simulink model "adc16_mytest"  (R2017a)
settings: Solver=VariableStepDiscrete  StartTime=0.0  StopTime=10.0  RelTol=1e-3
libraries: xbsIndex_r4 x3925, casper_library_misc x8, xps_library x1
(part 1 of 43)
settings Model: Creator=gopal  LastModifiedBy=root
settings DataIOCC: LimitDataPoints=on  SaveFormat=Array
settings OptimizationCC: DefaultParameterBehavior=Inlined  ExpressionDepthLimit=2147483647  LifeSpan=inf
settings DebuggingCC: UnderspecifiedInitializationDetection=Classic  MergeDetectMultiDrivingBlocksExec=none  SolverPrmCheckMsg=warning  StateNameClashWarn=warning  SFUnexpectedBacktrackingDiag=warning  SFNoUnconditionalDefaultTransitionDiag=warning  SFExecutionAtInitializationDiag=none
settings HardwareCC: ProdBitPerPointer=32  ProdBitPerSizeT=32  ProdBitPerPtrDiffT=32  ProdLargestAtomicFloat=None  ProdIntDivRoundTo=Undefined  ProdEndianess=Unspecified  ProdWordSize=32  ProdHWDeviceType=32-bit Generic
settings ModelReferenceCC: PropagateSignalLabelsOutOfModel=off
settings GRTTargetCC: TargetLangStandard=C89/C90 (ANSI)  GeneratePreprocessorConditionals=Disable all
settings ConfigComp: CovMetricSettings=dw  CovHtmlReporting=on  CovSaveCumulativeToWorkspaceVar=on  CovSaveSingleToWorkspaceVar=on  CovExternalEMLEnable=off

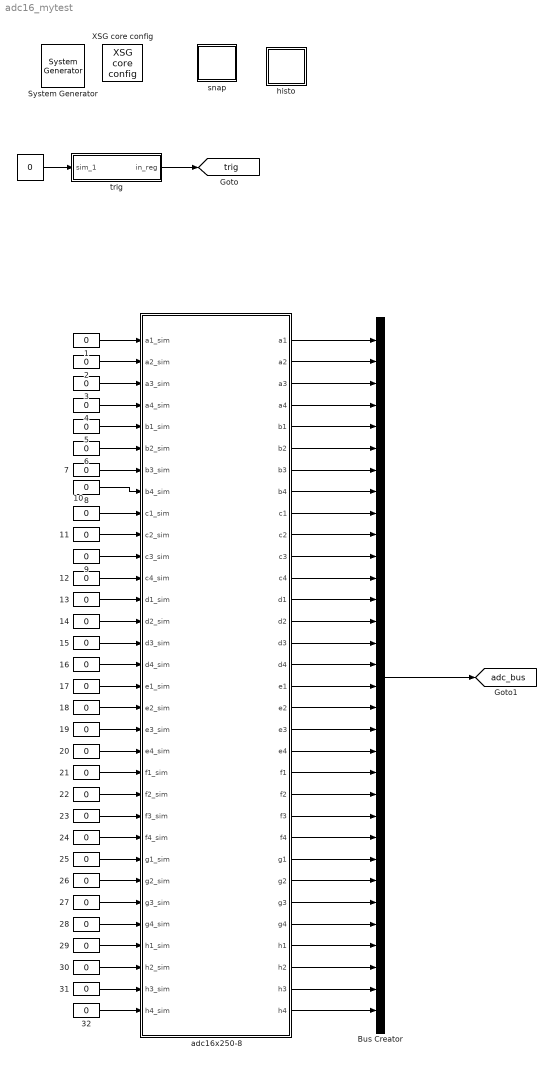
== system adc16_mytest ==
   {,1..32} (33 alike) : Constant  Value=0
  " System Generator" : xbsIndex_r4/ System Generator  Tag=genX  xilinxfamily=virtex6  part=xc6vsx475t  speed=-1  package=ff1759  synthesis_tool=XST  clock_wrapper=Clock Enables  directory=./adc16_mytest/sysgen  proj_type=Project Navigator  Synth_file=XST Defaults  Impl_file=ISE Defaults  testbench=off  simulink_period=1  sysclk_period=4.4444  dcm_input_clock_period=100  incr_netlist=off  trim_vbits=Everywhere in SubSystem  dbl_ovrd=According to Block Masks  core_generation=According to Block Masks  run_coregen=off  deprecated_control=off  eval_field=0  block_type=sysgen
  Bus Creator : BusCreator  Inputs=32
  XSG core config : xps_library/XSG core config  Tag=xps:xsg  hw_sys=ROACH2:sx475t  clk_src=adc0_clk  ROACH_clk_src=sys_clk  ROACH2_clk_src=adc0_clk  MKDIG_clk_src=sys_clk  clk_rate=225  sample_period=1  synthesis_tool=XST
      settings: SourceProductName=CASPER XPS Blockset
  adc16x250-8 : Subsystem  Tag=xps:adc16  AncestorBlock=xps_library/ADCs/adc16x250-8  mask(ADC16){board_count=2, roach2_rev=2, zdok_rev=2}
      mask prompts: board_count "Number of ADC16 Boards"; roach2_rev "ROACH2 Revision"; zdok_rev "ZDOK Pinout Revision"
      mask help: 16-input ADC. When using one ADC16 board, it must be in ZDOK0.
      mask init:
      | % Only board_count is needed by init function
      | adc16_init(gcb, ...
      |     'board_count', board_count);
      settings: AttributesFormatString=r2 rev%<roach2_rev>\nzdok rev%<zdok_rev>
      mask Help:
      | This is the CASPER "yellow block" for the CASPER ADC16 board.  Each ADC
      | board has four ADC chips.  Each ADC chip accepts four inputs.  The four
      | 8-bit outputs from each ADC chip are concatenated into a 32-bit signal.
      mask TypeOptions board_count: 1 | 2
      mask TypeOptions roach2_rev: 1 | 2
      mask TypeOptions zdok_rev: 1 | 2
  histo : Subsystem
  snap : Subsystem
  trig : Subsystem  Tag=xps:sw_reg  AncestorBlock=xps_library/software register  mask(swreg){mode=one value, io_dir=From Processor, io_delay=0, sample_period=1, names=reg, bitwidths=32, arith_types=0, bin_pts=0, sim_port=on, show_format=off}
      mask prompts: io_dir "I/O direction"; io_delay "I/O delay"; sample_period "Sample period"; names "Name:"; bitwidths "Bitwidth:"; arith_types "Type (ufix=0, fix=1, bool=2):"; bin_pts "Binary pt:"; sim_port "Provide sim input/output?"; show_format "Print format string?"
      mask init:
      | swreg_init(gcb)
      settings: AttributesFormatString=1input
      mask TypeOptions mode: one value | fields of equal size | fields of arbitrary size
      mask Callback mode: swreg_cb(gcb);
      mask TypeOptions io_dir: To Processor | From Processor
      mask Callback io_dir:
      | mask_enables = get_param(gcb, 'MaskEnables');
      | mask_names = get_param(gcb, 'MaskNames');
      | if strcmp(get_param(gcb, 'io_dir'), 'To Processor'),
      |     mask_enables{ismember(mask_names, 'sample_period')} = 'off';
      | else
      |     mask_enables{ismember(mask_names, 'sample_period')} = 'on';
      | end
      | set_param(gcb, 'MaskEnables', mask_enables);
      mask Callback bitwidths: swreg_maskcheck(gcb);
      mask Callback arith_types: [numios, ~, ~, ~, current_types] = swreg_maskcheck(gcb);
      mask Callback bin_pts: swreg_maskcheck(gcb);
  tag scope: adc_bus=global, trig=global
  wires:
  " "/1 -> trig/1(sim_1)
  trig/1(in_reg) -> [trig]
  " 1"/1 -> adc16x250-8/1(a1_sim)
  " 13"/1 -> adc16x250-8/13(d1_sim)
  " 4"/1 -> adc16x250-8/4(a4_sim)
  " 12"/1 -> adc16x250-8/12(c4_sim)
  " 6"/1 -> adc16x250-8/6(b2_sim)
  " 2"/1 -> adc16x250-8/2(a2_sim)
  " 15"/1 -> adc16x250-8/15(d3_sim)
  " 9"/1 -> adc16x250-8/11(c3_sim)
  " 5"/1 -> adc16x250-8/5(b1_sim)
  " 16"/1 -> adc16x250-8/16(d4_sim)
  " 7"/1 -> adc16x250-8/7(b3_sim)
  " 11"/1 -> adc16x250-8/10(c2_sim)
  " 10"/1 -> adc16x250-8/9(c1_sim)
  " 14"/1 -> adc16x250-8/14(d2_sim)
  " 29"/1 -> adc16x250-8/29(h1_sim)
  " 27"/1 -> adc16x250-8/27(g3_sim)
  " 18"/1 -> adc16x250-8/18(e2_sim)
  " 17"/1 -> adc16x250-8/17(e1_sim)
  " 19"/1 -> adc16x250-8/19(e3_sim)
  " 26"/1 -> adc16x250-8/26(g2_sim)
  " 20"/1 -> adc16x250-8/20(e4_sim)
  " 21"/1 -> adc16x250-8/21(f1_sim)
  " 24"/1 -> adc16x250-8/24(f4_sim)
  " 28"/1 -> adc16x250-8/28(g4_sim)
  " 23"/1 -> adc16x250-8/23(f3_sim)
  " 22"/1 -> adc16x250-8/22(f2_sim)
  " 31"/1 -> adc16x250-8/31(h3_sim)
  " 25"/1 -> adc16x250-8/25(g1_sim)
  " 30"/1 -> adc16x250-8/30(h2_sim)
  " 32"/1 -> adc16x250-8/32(h4_sim)
  " 3"/1 -> adc16x250-8/3(a3_sim)
  " 8"/1 -> adc16x250-8/8(b4_sim)
  adc16x250-8/14(d2) -> Bus Creator/14
  adc16x250-8/15(d3) -> Bus Creator/15
  adc16x250-8/16(d4) -> Bus Creator/16
  adc16x250-8/10(c2) -> Bus Creator/10
  adc16x250-8/1(a1) -> Bus Creator/1
  adc16x250-8/2(a2) -> Bus Creator/2
  adc16x250-8/3(a3) -> Bus Creator/3
  adc16x250-8/4(a4) -> Bus Creator/4
  adc16x250-8/5(b1) -> Bus Creator/5
  adc16x250-8/6(b2) -> Bus Creator/6
  adc16x250-8/7(b3) -> Bus Creator/7
  adc16x250-8/8(b4) -> Bus Creator/8
  adc16x250-8/9(c1) -> Bus Creator/9
  adc16x250-8/11(c3) -> Bus Creator/11
  adc16x250-8/12(c4) -> Bus Creator/12
  adc16x250-8/13(d1) -> Bus Creator/13
  adc16x250-8/22(f2) -> Bus Creator/22
  adc16x250-8/20(e4) -> Bus Creator/20
  adc16x250-8/21(f1) -> Bus Creator/21
  adc16x250-8/19(e3) -> Bus Creator/19
  adc16x250-8/25(g1) -> Bus Creator/25
  adc16x250-8/23(f3) -> Bus Creator/23
  adc16x250-8/18(e2) -> Bus Creator/18
  adc16x250-8/17(e1) -> Bus Creator/17
  adc16x250-8/24(f4) -> Bus Creator/24
  adc16x250-8/26(g2) -> Bus Creator/26
  adc16x250-8/27(g3) -> Bus Creator/27
  adc16x250-8/28(g4) -> Bus Creator/28
  adc16x250-8/29(h1) -> Bus Creator/29
  adc16x250-8/32(h4) -> Bus Creator/32
  adc16x250-8/30(h2) -> Bus Creator/30
  adc16x250-8/31(h3) -> Bus Creator/31
  Bus Creator/1 -> [adc_bus]

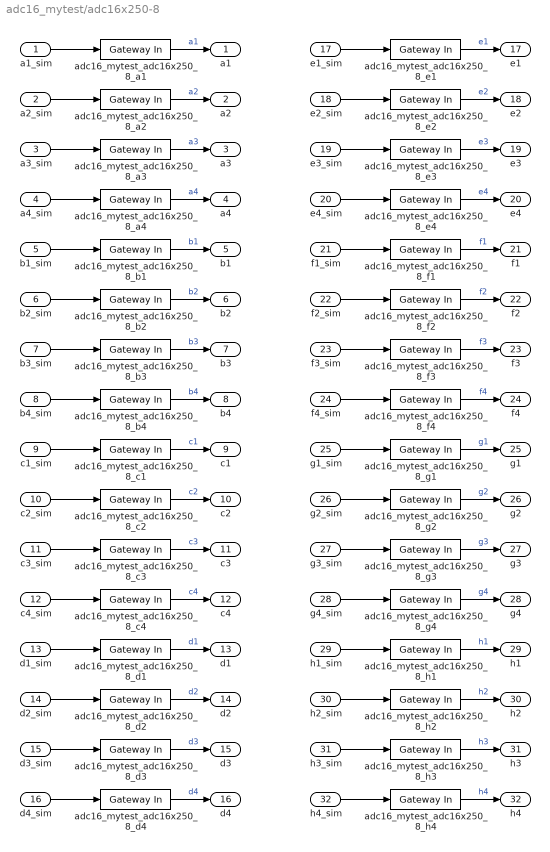
== system adc16_mytest/adc16x250-8 ==
  a1_sim : Inport
  a2_sim : Inport  Port=2
  a3_sim : Inport  Port=3
  a4_sim : Inport  Port=4
  b1_sim : Inport  Port=5
  b2_sim : Inport  Port=6
  b3_sim : Inport  Port=7
  b4_sim : Inport  Port=8
  c1_sim : Inport  Port=9
  c2_sim : Inport  Port=10
  c3_sim : Inport  Port=11
  c4_sim : Inport  Port=12
  d1_sim : Inport  Port=13
  d2_sim : Inport  Port=14
  d3_sim : Inport  Port=15
  d4_sim : Inport  Port=16
  e1_sim : Inport  Port=17
  e2_sim : Inport  Port=18
  e3_sim : Inport  Port=19
  e4_sim : Inport  Port=20
  f1_sim : Inport  Port=21
  f2_sim : Inport  Port=22
  f3_sim : Inport  Port=23
  f4_sim : Inport  Port=24
  g1_sim : Inport  Port=25
  g2_sim : Inport  Port=26
  g3_sim : Inport  Port=27
  g4_sim : Inport  Port=28
  h1_sim : Inport  Port=29
  h2_sim : Inport  Port=30
  h3_sim : Inport  Port=31
  h4_sim : Inport  Port=32
  adc16_mytest_adc16x250_8_a{1..4} (4 alike) : xbsIndex_r4/Gateway In  gui_display_data_type=Fixed-point  arith_type="Signed  (2's comp)"  n_bits=8  bin_pt=7  preci_type=Single  exp_width=8  frac_width=24  quantization="Round  (unbiased: +/- Inf)"  overflow=Saturate  period=1  dbl_ovrd=off  timing_constraint=None  locs_specified=off  LOCs={}  UseAsADC=off  ADCChannel='1'  inherit_from_input=off  hdl_port=on  block_type=gatewayin
  adc16_mytest_adc16x250_8_b{1..4} (4 alike) : xbsIndex_r4/Gateway In  gui_display_data_type=Fixed-point  arith_type="Signed  (2's comp)"  n_bits=8  bin_pt=7  preci_type=Single  exp_width=8  frac_width=24  quantization="Round  (unbiased: +/- Inf)"  overflow=Saturate  period=1  dbl_ovrd=off  timing_constraint=None  locs_specified=off  LOCs={}  UseAsADC=off  ADCChannel='1'  inherit_from_input=off  hdl_port=on  block_type=gatewayin
  adc16_mytest_adc16x250_8_c{1..4} (4 alike) : xbsIndex_r4/Gateway In  gui_display_data_type=Fixed-point  arith_type="Signed  (2's comp)"  n_bits=8  bin_pt=7  preci_type=Single  exp_width=8  frac_width=24  quantization="Round  (unbiased: +/- Inf)"  overflow=Saturate  period=1  dbl_ovrd=off  timing_constraint=None  locs_specified=off  LOCs={}  UseAsADC=off  ADCChannel='1'  inherit_from_input=off  hdl_port=on  block_type=gatewayin
  adc16_mytest_adc16x250_8_d{1..4} (4 alike) : xbsIndex_r4/Gateway In  gui_display_data_type=Fixed-point  arith_type="Signed  (2's comp)"  n_bits=8  bin_pt=7  preci_type=Single  exp_width=8  frac_width=24  quantization="Round  (unbiased: +/- Inf)"  overflow=Saturate  period=1  dbl_ovrd=off  timing_constraint=None  locs_specified=off  LOCs={}  UseAsADC=off  ADCChannel='1'  inherit_from_input=off  hdl_port=on  block_type=gatewayin
  adc16_mytest_adc16x250_8_e{1..4} (4 alike) : xbsIndex_r4/Gateway In  gui_display_data_type=Fixed-point  arith_type="Signed  (2's comp)"  n_bits=8  bin_pt=7  preci_type=Single  exp_width=8  frac_width=24  quantization="Round  (unbiased: +/- Inf)"  overflow=Saturate  period=1  dbl_ovrd=off  timing_constraint=None  locs_specified=off  LOCs={}  UseAsADC=off  ADCChannel='1'  inherit_from_input=off  hdl_port=on  block_type=gatewayin
  adc16_mytest_adc16x250_8_f{1..4} (4 alike) : xbsIndex_r4/Gateway In  gui_display_data_type=Fixed-point  arith_type="Signed  (2's comp)"  n_bits=8  bin_pt=7  preci_type=Single  exp_width=8  frac_width=24  quantization="Round  (unbiased: +/- Inf)"  overflow=Saturate  period=1  dbl_ovrd=off  timing_constraint=None  locs_specified=off  LOCs={}  UseAsADC=off  ADCChannel='1'  inherit_from_input=off  hdl_port=on  block_type=gatewayin
  adc16_mytest_adc16x250_8_g{1..4} (4 alike) : xbsIndex_r4/Gateway In  gui_display_data_type=Fixed-point  arith_type="Signed  (2's comp)"  n_bits=8  bin_pt=7  preci_type=Single  exp_width=8  frac_width=24  quantization="Round  (unbiased: +/- Inf)"  overflow=Saturate  period=1  dbl_ovrd=off  timing_constraint=None  locs_specified=off  LOCs={}  UseAsADC=off  ADCChannel='1'  inherit_from_input=off  hdl_port=on  block_type=gatewayin
  adc16_mytest_adc16x250_8_h{1..4} (4 alike) : xbsIndex_r4/Gateway In  gui_display_data_type=Fixed-point  arith_type="Signed  (2's comp)"  n_bits=8  bin_pt=7  preci_type=Single  exp_width=8  frac_width=24  quantization="Round  (unbiased: +/- Inf)"  overflow=Saturate  period=1  dbl_ovrd=off  timing_constraint=None  locs_specified=off  LOCs={}  UseAsADC=off  ADCChannel='1'  inherit_from_input=off  hdl_port=on  block_type=gatewayin
  a1 : Outport
  a2 : Outport  Port=2
  a3 : Outport  Port=3
  a4 : Outport  Port=4
  b1 : Outport  Port=5
  b2 : Outport  Port=6
  b3 : Outport  Port=7
  b4 : Outport  Port=8
  c1 : Outport  Port=9
  c2 : Outport  Port=10
  c3 : Outport  Port=11
  c4 : Outport  Port=12
  d1 : Outport  Port=13
  d2 : Outport  Port=14
  d3 : Outport  Port=15
  d4 : Outport  Port=16
  e1 : Outport  Port=17
  e2 : Outport  Port=18
  e3 : Outport  Port=19
  e4 : Outport  Port=20
  f1 : Outport  Port=21
  f2 : Outport  Port=22
  f3 : Outport  Port=23
  f4 : Outport  Port=24
  g1 : Outport  Port=25
  g2 : Outport  Port=26
  g3 : Outport  Port=27
  g4 : Outport  Port=28
  h1 : Outport  Port=29
  h2 : Outport  Port=30
  h3 : Outport  Port=31
  h4 : Outport  Port=32
  wires:
  a1_sim/1 -> adc16_mytest_adc16x250_8_a1/1
  adc16_mytest_adc16x250_8_a1/1 -> a1/1  "a1"
  a2_sim/1 -> adc16_mytest_adc16x250_8_a2/1
  adc16_mytest_adc16x250_8_a2/1 -> a2/1  "a2"
  a3_sim/1 -> adc16_mytest_adc16x250_8_a3/1
  adc16_mytest_adc16x250_8_a3/1 -> a3/1  "a3"
  a4_sim/1 -> adc16_mytest_adc16x250_8_a4/1
  adc16_mytest_adc16x250_8_a4/1 -> a4/1  "a4"
  b1_sim/1 -> adc16_mytest_adc16x250_8_b1/1
  adc16_mytest_adc16x250_8_b1/1 -> b1/1  "b1"
  b2_sim/1 -> adc16_mytest_adc16x250_8_b2/1
  adc16_mytest_adc16x250_8_b2/1 -> b2/1  "b2"
  b3_sim/1 -> adc16_mytest_adc16x250_8_b3/1
  adc16_mytest_adc16x250_8_b3/1 -> b3/1  "b3"
  b4_sim/1 -> adc16_mytest_adc16x250_8_b4/1
  adc16_mytest_adc16x250_8_b4/1 -> b4/1  "b4"
  c1_sim/1 -> adc16_mytest_adc16x250_8_c1/1
  adc16_mytest_adc16x250_8_c1/1 -> c1/1  "c1"
  c2_sim/1 -> adc16_mytest_adc16x250_8_c2/1
  adc16_mytest_adc16x250_8_c2/1 -> c2/1  "c2"
  c3_sim/1 -> adc16_mytest_adc16x250_8_c3/1
  adc16_mytest_adc16x250_8_c3/1 -> c3/1  "c3"
  c4_sim/1 -> adc16_mytest_adc16x250_8_c4/1
  adc16_mytest_adc16x250_8_c4/1 -> c4/1  "c4"
  d1_sim/1 -> adc16_mytest_adc16x250_8_d1/1
  adc16_mytest_adc16x250_8_d1/1 -> d1/1  "d1"
  d2_sim/1 -> adc16_mytest_adc16x250_8_d2/1
  adc16_mytest_adc16x250_8_d2/1 -> d2/1  "d2"
  d3_sim/1 -> adc16_mytest_adc16x250_8_d3/1
  adc16_mytest_adc16x250_8_d3/1 -> d3/1  "d3"
  d4_sim/1 -> adc16_mytest_adc16x250_8_d4/1
  adc16_mytest_adc16x250_8_d4/1 -> d4/1  "d4"
  e1_sim/1 -> adc16_mytest_adc16x250_8_e1/1
  adc16_mytest_adc16x250_8_e1/1 -> e1/1  "e1"
  e2_sim/1 -> adc16_mytest_adc16x250_8_e2/1
  adc16_mytest_adc16x250_8_e2/1 -> e2/1  "e2"
  e3_sim/1 -> adc16_mytest_adc16x250_8_e3/1
  adc16_mytest_adc16x250_8_e3/1 -> e3/1  "e3"
  e4_sim/1 -> adc16_mytest_adc16x250_8_e4/1
  adc16_mytest_adc16x250_8_e4/1 -> e4/1  "e4"
  f1_sim/1 -> adc16_mytest_adc16x250_8_f1/1
  adc16_mytest_adc16x250_8_f1/1 -> f1/1  "f1"
  f2_sim/1 -> adc16_mytest_adc16x250_8_f2/1
  adc16_mytest_adc16x250_8_f2/1 -> f2/1  "f2"
  f3_sim/1 -> adc16_mytest_adc16x250_8_f3/1
  adc16_mytest_adc16x250_8_f3/1 -> f3/1  "f3"
  f4_sim/1 -> adc16_mytest_adc16x250_8_f4/1
  adc16_mytest_adc16x250_8_f4/1 -> f4/1  "f4"
  g1_sim/1 -> adc16_mytest_adc16x250_8_g1/1
  adc16_mytest_adc16x250_8_g1/1 -> g1/1  "g1"
  g2_sim/1 -> adc16_mytest_adc16x250_8_g2/1
  adc16_mytest_adc16x250_8_g2/1 -> g2/1  "g2"
  g3_sim/1 -> adc16_mytest_adc16x250_8_g3/1
  adc16_mytest_adc16x250_8_g3/1 -> g3/1  "g3"
  g4_sim/1 -> adc16_mytest_adc16x250_8_g4/1
  adc16_mytest_adc16x250_8_g4/1 -> g4/1  "g4"
  h1_sim/1 -> adc16_mytest_adc16x250_8_h1/1
  adc16_mytest_adc16x250_8_h1/1 -> h1/1  "h1"
  h2_sim/1 -> adc16_mytest_adc16x250_8_h2/1
  adc16_mytest_adc16x250_8_h2/1 -> h2/1  "h2"
  h3_sim/1 -> adc16_mytest_adc16x250_8_h3/1
  adc16_mytest_adc16x250_8_h3/1 -> h3/1  "h3"
  h4_sim/1 -> adc16_mytest_adc16x250_8_h4/1
  adc16_mytest_adc16x250_8_h4/1 -> h4/1  "h4"

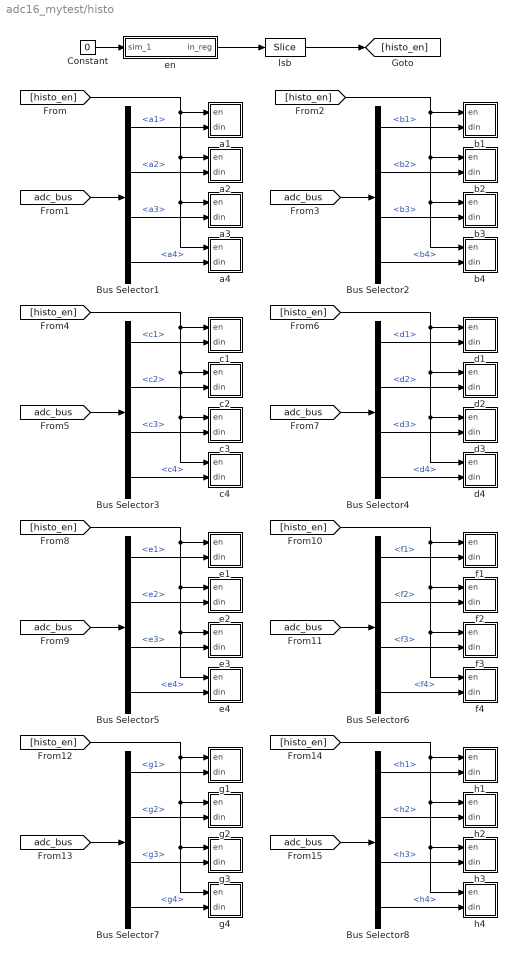
== system adc16_mytest/histo ==
  Bus Selector1 : BusSelector  OutputSignals=a1,a2,a3,a4
  Bus Selector2 : BusSelector  OutputSignals=b1,b2,b3,b4
  Bus Selector3 : BusSelector  OutputSignals=c1,c2,c3,c4
  Bus Selector4 : BusSelector  OutputSignals=d1,d2,d3,d4
  Bus Selector5 : BusSelector  OutputSignals=e1,e2,e3,e4
  Bus Selector6 : BusSelector  OutputSignals=f1,f2,f3,f4
  Bus Selector7 : BusSelector  OutputSignals=g1,g2,g3,g4
  Bus Selector8 : BusSelector  OutputSignals=h1,h2,h3,h4
  Constant : Constant  Value=0
  a1 : Subsystem
  a2 : Subsystem
  a3 : Subsystem
  a4 : Subsystem
  b1 : Subsystem
  b2 : Subsystem
  b3 : Subsystem
  b4 : Subsystem
  c1 : Subsystem
  c2 : Subsystem
  c3 : Subsystem
  c4 : Subsystem
  d1 : Subsystem
  d2 : Subsystem
  d3 : Subsystem
  d4 : Subsystem
  e1 : Subsystem
  e2 : Subsystem
  e3 : Subsystem
  e4 : Subsystem
  en : Subsystem  Tag=xps:sw_reg  AncestorBlock=xps_library/software register  mask(swreg){mode=one value, io_dir=From Processor, io_delay=0, sample_period=1, names=reg, bitwidths=32, arith_types=0, bin_pts=0, sim_port=on, show_format=off}
      mask prompts: io_dir "I/O direction"; io_delay "I/O delay"; sample_period "Sample period"; names "Name:"; bitwidths "Bitwidth:"; arith_types "Type (ufix=0, fix=1, bool=2):"; bin_pts "Binary pt:"; sim_port "Provide sim input/output?"; show_format "Print format string?"
      mask init:
      | swreg_init(gcb)
      settings: AttributesFormatString=1input
      mask TypeOptions mode: one value | fields of equal size | fields of arbitrary size
      mask Callback mode: swreg_cb(gcb);
      mask TypeOptions io_dir: To Processor | From Processor
      mask Callback io_dir:
      | mask_enables = get_param(gcb, 'MaskEnables');
      | mask_names = get_param(gcb, 'MaskNames');
      | if strcmp(get_param(gcb, 'io_dir'), 'To Processor'),
      |     mask_enables{ismember(mask_names, 'sample_period')} = 'off';
      | else
      |     mask_enables{ismember(mask_names, 'sample_period')} = 'on';
      | end
      | set_param(gcb, 'MaskEnables', mask_enables);
      mask Callback bitwidths: swreg_maskcheck(gcb);
      mask Callback arith_types: [numios, ~, ~, ~, current_types] = swreg_maskcheck(gcb);
      mask Callback bin_pts: swreg_maskcheck(gcb);
  f1 : Subsystem
  f2 : Subsystem
  f3 : Subsystem
  f4 : Subsystem
  g1 : Subsystem
  g2 : Subsystem
  g3 : Subsystem
  g4 : Subsystem
  h1 : Subsystem
  h2 : Subsystem
  h3 : Subsystem
  h4 : Subsystem
  lsb : xbsIndex_r4/Slice  nbits=1  boolean_output=on  mode=Lower Bit Location + Width  bit1=0  base1=MSB of Input  bit0=0  base0=LSB of Input  dbl_ovrd=off  block_type=slice
  wires:
  Bus Selector8/2 -> h2/2(din)  "<h2>"
  Bus Selector8/3 -> h3/2(din)  "<h3>"
  Bus Selector8/4 -> h4/2(din)  "<h4>"
  Bus Selector8/1 -> h1/2(din)  "<h1>"
  [histo_en] -> h1/1(en), h2/1(en), h3/1(en), h4/1(en)
  [adc_bus] -> Bus Selector8/1
  Bus Selector7/2 -> g2/2(din)  "<g2>"
  Bus Selector7/3 -> g3/2(din)  "<g3>"
  Bus Selector7/4 -> g4/2(din)  "<g4>"
  Bus Selector7/1 -> g1/2(din)  "<g1>"
  [histo_en] -> g1/1(en), g2/1(en), g3/1(en), g4/1(en)
  [adc_bus] -> Bus Selector7/1
  Bus Selector6/2 -> f2/2(din)  "<f2>"
  Bus Selector6/3 -> f3/2(din)  "<f3>"
  Bus Selector6/4 -> f4/2(din)  "<f4>"
  Bus Selector6/1 -> f1/2(din)  "<f1>"
  [histo_en] -> f1/1(en), f2/1(en), f3/1(en), f4/1(en)
  [adc_bus] -> Bus Selector6/1
  Bus Selector5/2 -> e2/2(din)  "<e2>"
  Bus Selector5/3 -> e3/2(din)  "<e3>"
  Bus Selector5/4 -> e4/2(din)  "<e4>"
  Bus Selector5/1 -> e1/2(din)  "<e1>"
  [histo_en] -> e1/1(en), e2/1(en), e3/1(en), e4/1(en)
  [adc_bus] -> Bus Selector5/1
  Bus Selector4/2 -> d2/2(din)  "<d2>"
  Bus Selector4/3 -> d3/2(din)  "<d3>"
  Bus Selector4/4 -> d4/2(din)  "<d4>"
  Bus Selector4/1 -> d1/2(din)  "<d1>"
  [histo_en] -> d1/1(en), d2/1(en), d3/1(en), d4/1(en)
  [adc_bus] -> Bus Selector4/1
  Bus Selector3/2 -> c2/2(din)  "<c2>"
  Bus Selector3/3 -> c3/2(din)  "<c3>"
  Bus Selector3/4 -> c4/2(din)  "<c4>"
  Bus Selector3/1 -> c1/2(din)  "<c1>"
  [histo_en] -> c1/1(en), c2/1(en), c3/1(en), c4/1(en)
  [adc_bus] -> Bus Selector3/1
  Bus Selector2/2 -> b2/2(din)  "<b2>"
  Bus Selector2/3 -> b3/2(din)  "<b3>"
  Bus Selector2/4 -> b4/2(din)  "<b4>"
  Bus Selector2/1 -> b1/2(din)  "<b1>"
  [histo_en] -> b1/1(en), b2/1(en), b3/1(en), b4/1(en)
  [adc_bus] -> Bus Selector2/1
  Bus Selector1/2 -> a2/2(din)  "<a2>"
  Bus Selector1/3 -> a3/2(din)  "<a3>"
  Bus Selector1/4 -> a4/2(din)  "<a4>"
  Bus Selector1/1 -> a1/2(din)  "<a1>"
  [histo_en] -> a1/1(en), a2/1(en), a3/1(en), a4/1(en)
  [adc_bus] -> Bus Selector1/1
  lsb/1 -> [histo_en]
  Constant/1 -> en/1(sim_1)
  en/1(in_reg) -> lsb/1

== system adc16_mytest/snap ==
  BitBasher : xbsIndex_r4/BitBasher  bitexpr=|  display_expr=off  sr_1=1  arith_type1=Unsigned  bin_pt1=0  sr_2=2  arith_type2=Unsigned  bin_pt2=0  sr_3=3  arith_type3=Unsigned  bin_pt3=0  sr_4=4  arith_type4=Unsigned  bin_pt4=0  dbl_ovrd=off  block_type=bitbasher
      | <!DOCTYPE HTML PUBLIC "-//W3C//DTD HTML 4.0//EN" "http://www.w3.org/TR/REC-html40/strict.dtd">
      | <html><head><meta name="qrichtext" content="1" /><style type="text/css">
      | p, li { white-space: pre-wrap; }
      | </style></head><body style=" font-family:'Sans'; font-size:10pt; font-weight:400; font-style:normal;">
      | <p style=" margin-top:12px; margin-bottom:12px; margin-left:0px; margin-right:0px; -qt-block-indent:0; text-indent:0px;"><span style=" font-family:'MS Shell Dlg'; font-size:8pt;">o={p1,p2,p3,p4}</span></p></body></html>
  BitBasher1 : xbsIndex_r4/BitBasher  bitexpr=|  display_expr=off  sr_1=1  arith_type1=Unsigned  bin_pt1=0  sr_2=2  arith_type2=Unsigned  bin_pt2=0  sr_3=3  arith_type3=Unsigned  bin_pt3=0  sr_4=4  arith_type4=Unsigned  bin_pt4=0  dbl_ovrd=off  block_type=bitbasher
      | <!DOCTYPE HTML PUBLIC "-//W3C//DTD HTML 4.0//EN" "http://www.w3.org/TR/REC-html40/strict.dtd">
      | <html><head><meta name="qrichtext" content="1" /><style type="text/css">
      | p, li { white-space: pre-wrap; }
      | </style></head><body style=" font-family:'Sans'; font-size:10pt; font-weight:400; font-style:normal;">
      | <p style=" margin-top:12px; margin-bottom:12px; margin-left:0px; margin-right:0px; -qt-block-indent:0; text-indent:0px;"><span style=" font-family:'MS Shell Dlg'; font-size:8pt;">o={p1,p2,p3,p4}</span></p></body></html>
  BitBasher10 : xbsIndex_r4/BitBasher  bitexpr=|  display_expr=off  sr_1=1  arith_type1=Unsigned  bin_pt1=0  sr_2=2  arith_type2=Unsigned  bin_pt2=0  sr_3=3  arith_type3=Unsigned  bin_pt3=0  sr_4=4  arith_type4=Unsigned  bin_pt4=0  dbl_ovrd=off  block_type=bitbasher
      | <!DOCTYPE HTML PUBLIC "-//W3C//DTD HTML 4.0//EN" "http://www.w3.org/TR/REC-html40/strict.dtd">
      | <html><head><meta name="qrichtext" content="1" /><style type="text/css">
      | p, li { white-space: pre-wrap; }
      | </style></head><body style=" font-family:'Sans'; font-size:10pt; font-weight:400; font-style:normal;">
      | <p style=" margin-top:12px; margin-bottom:12px; margin-left:0px; margin-right:0px; -qt-block-indent:0; text-indent:0px;"><span style=" font-family:'MS Shell Dlg'; font-size:8pt;">o={p1,p2,p3,p4}</span></p></body></html>
  BitBasher11 : xbsIndex_r4/BitBasher  bitexpr=|  display_expr=off  sr_1=1  arith_type1=Unsigned  bin_pt1=0  sr_2=2  arith_type2=Unsigned  bin_pt2=0  sr_3=3  arith_type3=Unsigned  bin_pt3=0  sr_4=4  arith_type4=Unsigned  bin_pt4=0  dbl_ovrd=off  block_type=bitbasher
      | <!DOCTYPE HTML PUBLIC "-//W3C//DTD HTML 4.0//EN" "http://www.w3.org/TR/REC-html40/strict.dtd">
      | <html><head><meta name="qrichtext" content="1" /><style type="text/css">
      | p, li { white-space: pre-wrap; }
      | </style></head><body style=" font-family:'Sans'; font-size:10pt; font-weight:400; font-style:normal;">
      | <p style=" margin-top:12px; margin-bottom:12px; margin-left:0px; margin-right:0px; -qt-block-indent:0; text-indent:0px;"><span style=" font-family:'MS Shell Dlg'; font-size:8pt;">o={p1,p2,p3,p4}</span></p></body></html>
  BitBasher2 : xbsIndex_r4/BitBasher  bitexpr=|  display_expr=off  sr_1=1  arith_type1=Unsigned  bin_pt1=0  sr_2=2  arith_type2=Unsigned  bin_pt2=0  sr_3=3  arith_type3=Unsigned  bin_pt3=0  sr_4=4  arith_type4=Unsigned  bin_pt4=0  dbl_ovrd=off  block_type=bitbasher
      | <!DOCTYPE HTML PUBLIC "-//W3C//DTD HTML 4.0//EN" "http://www.w3.org/TR/REC-html40/strict.dtd">
      | <html><head><meta name="qrichtext" content="1" /><style type="text/css">
      | p, li { white-space: pre-wrap; }
      | </style></head><body style=" font-family:'Sans'; font-size:10pt; font-weight:400; font-style:normal;">
      | <p style=" margin-top:12px; margin-bottom:12px; margin-left:0px; margin-right:0px; -qt-block-indent:0; text-indent:0px;"><span style=" font-family:'MS Shell Dlg'; font-size:8pt;">o={p1,p2,p3,p4}</span></p></body></html>
  BitBasher3 : xbsIndex_r4/BitBasher  bitexpr=|  display_expr=off  sr_1=1  arith_type1=Unsigned  bin_pt1=0  sr_2=2  arith_type2=Unsigned  bin_pt2=0  sr_3=3  arith_type3=Unsigned  bin_pt3=0  sr_4=4  arith_type4=Unsigned  bin_pt4=0  dbl_ovrd=off  block_type=bitbasher
      | <!DOCTYPE HTML PUBLIC "-//W3C//DTD HTML 4.0//EN" "http://www.w3.org/TR/REC-html40/strict.dtd">
      | <html><head><meta name="qrichtext" content="1" /><style type="text/css">
      | p, li { white-space: pre-wrap; }
      | </style></head><body style=" font-family:'Sans'; font-size:10pt; font-weight:400; font-style:normal;">
      | <p style=" margin-top:12px; margin-bottom:12px; margin-left:0px; margin-right:0px; -qt-block-indent:0; text-indent:0px;"><span style=" font-family:'MS Shell Dlg'; font-size:8pt;">o={p1,p2,p3,p4}</span></p></body></html>
  BitBasher8 : xbsIndex_r4/BitBasher  bitexpr=|  display_expr=off  sr_1=1  arith_type1=Unsigned  bin_pt1=0  sr_2=2  arith_type2=Unsigned  bin_pt2=0  sr_3=3  arith_type3=Unsigned  bin_pt3=0  sr_4=4  arith_type4=Unsigned  bin_pt4=0  dbl_ovrd=off  block_type=bitbasher
      | <!DOCTYPE HTML PUBLIC "-//W3C//DTD HTML 4.0//EN" "http://www.w3.org/TR/REC-html40/strict.dtd">
      | <html><head><meta name="qrichtext" content="1" /><style type="text/css">
      | p, li { white-space: pre-wrap; }
      | </style></head><body style=" font-family:'Sans'; font-size:10pt; font-weight:400; font-style:normal;">
      | <p style=" margin-top:12px; margin-bottom:12px; margin-left:0px; margin-right:0px; -qt-block-indent:0; text-indent:0px;"><span style=" font-family:'MS Shell Dlg'; font-size:8pt;">o={p1,p2,p3,p4}</span></p></body></html>
  BitBasher9 : xbsIndex_r4/BitBasher  bitexpr=|  display_expr=off  sr_1=1  arith_type1=Unsigned  bin_pt1=0  sr_2=2  arith_type2=Unsigned  bin_pt2=0  sr_3=3  arith_type3=Unsigned  bin_pt3=0  sr_4=4  arith_type4=Unsigned  bin_pt4=0  dbl_ovrd=off  block_type=bitbasher
      | <!DOCTYPE HTML PUBLIC "-//W3C//DTD HTML 4.0//EN" "http://www.w3.org/TR/REC-html40/strict.dtd">
      | <html><head><meta name="qrichtext" content="1" /><style type="text/css">
      | p, li { white-space: pre-wrap; }
      | </style></head><body style=" font-family:'Sans'; font-size:10pt; font-weight:400; font-style:normal;">
      | <p style=" margin-top:12px; margin-bottom:12px; margin-left:0px; margin-right:0px; -qt-block-indent:0; text-indent:0px;"><span style=" font-family:'MS Shell Dlg'; font-size:8pt;">o={p1,p2,p3,p4}</span></p></body></html>
  Bus Selector : BusSelector  OutputSignals=a1,a2,a3,a4,b1,b2,b3,b4,c1,c2,c3,c4,d1,d2,d3,d4
  Bus Selector2 : BusSelector  OutputSignals=e1,e2,e3,e4,f1,f2,f3,f4,g1,g2,g3,g4,h1,h2,h3,h4
  Constant1 : xbsIndex_r4/Constant  const=0  gui_display_data_type=Boolean  arith_type=Boolean  n_bits=16  bin_pt=14  preci_type=Single  exp_width=8  frac_width=24  explicit_period=on  period=1  equ=P=C  opselect=C  inp2=PCIN>>17  opr=+  inp1=P  carry=CIN  dbl_ovrd=off  block_type=constant
  Constant2 : xbsIndex_r4/Constant  const=0  gui_display_data_type=Boolean  arith_type=Boolean  n_bits=16  bin_pt=14  preci_type=Single  exp_width=8  frac_width=24  explicit_period=on  period=1  equ=P=C  opselect=C  inp2=PCIN>>17  opr=+  inp1=P  carry=CIN  dbl_ovrd=off  block_type=constant
  Slice : xbsIndex_r4/Slice  nbits=1  boolean_output=on  mode=Lower Bit Location + Width  bit1=0  base1=MSB of Input  bit0=0  base0=LSB of Input  dbl_ovrd=off  block_type=slice
  a : Subsystem  Tag=casper:snapshot  AncestorBlock=casper_library_scopes/snapshot  mask(snapshot){storage=bram, dram_dimm=1, dram_clock=200, nsamples=10, data_width=32, offset=off, circap=off, value=off, use_dsp48=off}
      mask prompts: storage "Storage medium"; dram_dimm "DRAM dimm"; dram_clock "DRAM clock rate"; nsamples "Number of Samples (2^?)"; data_width "Data width"; offset "Start delay support"; circap "Circular capture support"; value "Extra value capture support"; use_dsp48 "Use DSP48s to implement counters"
      mask help:
      | Standard snap block, but with the following optional extras;
      |  1) Optionally delay the fabric trigger by a user-specified number of valids.
      |  2) Capture continuously after a trigger until a stop pulse is received. Data is captured into BRAM continuously, with old data being overwritten until a stop command is received. Then stop capturing when memory is filled. This enables you to get some data before and some data after the stop pulse. Use the 'tr_en_cnt' register to determine where you are in your vector. 'Addr' register's MSb now indicates 'busy capturing'.
      |  3) Optionally capture a value on an input port to a register at the same time as the first data sample.
      |  4) Implement counters using DSP48Es to save resources.
      mask init:
      | snapshot_init(gcb, ...
      |     'storage', storage, ...
      |     'dram_dimm', dram_dimm, ...
      |     'dram_clock', dram_clock, ...
      |     'nsamples', nsamples, ...
      |     'data_width', data_width, ...
      |     'offset', offset, ...
      |     'circap', circap, ...
      |     'value', value, ...
      |     'use_dsp48', use_dsp48);
      mask TypeOptions storage: bram | dram
      mask Callback storage: snapshot_callback();
      mask TypeOptions dram_dimm: 1 | 2 | 3 | 4
      mask TypeOptions dram_clock: 200 | 250 | 266 | 300 | 333
      mask TypeOptions data_width: 8 | 16 | 32 | 64 | 128
  b : Subsystem  Tag=casper:snapshot  AncestorBlock=casper_library_scopes/snapshot  mask(snapshot){storage=bram, dram_dimm=1, dram_clock=200, nsamples=10, data_width=32, offset=off, circap=off, value=off, use_dsp48=off}
      mask prompts: storage "Storage medium"; dram_dimm "DRAM dimm"; dram_clock "DRAM clock rate"; nsamples "Number of Samples (2^?)"; data_width "Data width"; offset "Start delay support"; circap "Circular capture support"; value "Extra value capture support"; use_dsp48 "Use DSP48s to implement counters"
      mask help:
      | Standard snap block, but with the following optional extras;
      |  1) Optionally delay the fabric trigger by a user-specified number of valids.
      |  2) Capture continuously after a trigger until a stop pulse is received. Data is captured into BRAM continuously, with old data being overwritten until a stop command is received. Then stop capturing when memory is filled. This enables you to get some data before and some data after the stop pulse. Use the 'tr_en_cnt' register to determine where you are in your vector. 'Addr' register's MSb now indicates 'busy capturing'.
      |  3) Optionally capture a value on an input port to a register at the same time as the first data sample.
      |  4) Implement counters using DSP48Es to save resources.
      mask init: same as adc16_mytest/snap/a
      mask TypeOptions storage: bram | dram
      mask Callback storage: snapshot_callback();
      mask TypeOptions dram_dimm: 1 | 2 | 3 | 4
      mask TypeOptions dram_clock: 200 | 250 | 266 | 300 | 333
      mask TypeOptions data_width: 8 | 16 | 32 | 64 | 128
  c : Subsystem  Tag=casper:snapshot  AncestorBlock=casper_library_scopes/snapshot  mask(snapshot){storage=bram, dram_dimm=1, dram_clock=200, nsamples=10, data_width=32, offset=off, circap=off, value=off, use_dsp48=off}
      mask prompts: storage "Storage medium"; dram_dimm "DRAM dimm"; dram_clock "DRAM clock rate"; nsamples "Number of Samples (2^?)"; data_width "Data width"; offset "Start delay support"; circap "Circular capture support"; value "Extra value capture support"; use_dsp48 "Use DSP48s to implement counters"
      mask help:
      | Standard snap block, but with the following optional extras;
      |  1) Optionally delay the fabric trigger by a user-specified number of valids.
      |  2) Capture continuously after a trigger until a stop pulse is received. Data is captured into BRAM continuously, with old data being overwritten until a stop command is received. Then stop capturing when memory is filled. This enables you to get some data before and some data after the stop pulse. Use the 'tr_en_cnt' register to determine where you are in your vector. 'Addr' register's MSb now indicates 'busy capturing'.
      |  3) Optionally capture a value on an input port to a register at the same time as the first data sample.
      |  4) Implement counters using DSP48Es to save resources.
      mask init: same as adc16_mytest/snap/a
      mask TypeOptions storage: bram | dram
      mask Callback storage: snapshot_callback();
      mask TypeOptions dram_dimm: 1 | 2 | 3 | 4
      mask TypeOptions dram_clock: 200 | 250 | 266 | 300 | 333
      mask TypeOptions data_width: 8 | 16 | 32 | 64 | 128
  d : Subsystem  Tag=casper:snapshot  AncestorBlock=casper_library_scopes/snapshot  mask(snapshot){storage=bram, dram_dimm=1, dram_clock=200, nsamples=10, data_width=32, offset=off, circap=off, value=off, use_dsp48=off}
      mask prompts: storage "Storage medium"; dram_dimm "DRAM dimm"; dram_clock "DRAM clock rate"; nsamples "Number of Samples (2^?)"; data_width "Data width"; offset "Start delay support"; circap "Circular capture support"; value "Extra value capture support"; use_dsp48 "Use DSP48s to implement counters"
      mask help:
      | Standard snap block, but with the following optional extras;
      |  1) Optionally delay the fabric trigger by a user-specified number of valids.
      |  2) Capture continuously after a trigger until a stop pulse is received. Data is captured into BRAM continuously, with old data being overwritten until a stop command is received. Then stop capturing when memory is filled. This enables you to get some data before and some data after the stop pulse. Use the 'tr_en_cnt' register to determine where you are in your vector. 'Addr' register's MSb now indicates 'busy capturing'.
      |  3) Optionally capture a value on an input port to a register at the same time as the first data sample.
      |  4) Implement counters using DSP48Es to save resources.
      mask init: same as adc16_mytest/snap/a
      mask TypeOptions storage: bram | dram
      mask Callback storage: snapshot_callback();
      mask TypeOptions dram_dimm: 1 | 2 | 3 | 4
      mask TypeOptions dram_clock: 200 | 250 | 266 | 300 | 333
      mask TypeOptions data_width: 8 | 16 | 32 | 64 | 128
  e : Subsystem  Tag=casper:snapshot  AncestorBlock=casper_library_scopes/snapshot  mask(snapshot){storage=bram, dram_dimm=1, dram_clock=200, nsamples=10, data_width=32, offset=off, circap=off, value=off, use_dsp48=off}
      mask prompts: storage "Storage medium"; dram_dimm "DRAM dimm"; dram_clock "DRAM clock rate"; nsamples "Number of Samples (2^?)"; data_width "Data width"; offset "Start delay support"; circap "Circular capture support"; value "Extra value capture support"; use_dsp48 "Use DSP48s to implement counters"
      mask help:
      | Standard snap block, but with the following optional extras;
      |  1) Optionally delay the fabric trigger by a user-specified number of valids.
      |  2) Capture continuously after a trigger until a stop pulse is received. Data is captured into BRAM continuously, with old data being overwritten until a stop command is received. Then stop capturing when memory is filled. This enables you to get some data before and some data after the stop pulse. Use the 'tr_en_cnt' register to determine where you are in your vector. 'Addr' register's MSb now indicates 'busy capturing'.
      |  3) Optionally capture a value on an input port to a register at the same time as the first data sample.
      |  4) Implement counters using DSP48Es to save resources.
      mask init: same as adc16_mytest/snap/a
      mask TypeOptions storage: bram | dram
      mask Callback storage: snapshot_callback();
      mask TypeOptions dram_dimm: 1 | 2 | 3 | 4
      mask TypeOptions dram_clock: 200 | 250 | 266 | 300 | 333
      mask TypeOptions data_width: 8 | 16 | 32 | 64 | 128
  f : Subsystem  Tag=casper:snapshot  AncestorBlock=casper_library_scopes/snapshot  mask(snapshot){storage=bram, dram_dimm=1, dram_clock=200, nsamples=10, data_width=32, offset=off, circap=off, value=off, use_dsp48=off}
      mask prompts: storage "Storage medium"; dram_dimm "DRAM dimm"; dram_clock "DRAM clock rate"; nsamples "Number of Samples (2^?)"; data_width "Data width"; offset "Start delay support"; circap "Circular capture support"; value "Extra value capture support"; use_dsp48 "Use DSP48s to implement counters"
      mask help:
      | Standard snap block, but with the following optional extras;
      |  1) Optionally delay the fabric trigger by a user-specified number of valids.
      |  2) Capture continuously after a trigger until a stop pulse is received. Data is captured into BRAM continuously, with old data being overwritten until a stop command is received. Then stop capturing when memory is filled. This enables you to get some data before and some data after the stop pulse. Use the 'tr_en_cnt' register to determine where you are in your vector. 'Addr' register's MSb now indicates 'busy capturing'.
      |  3) Optionally capture a value on an input port to a register at the same time as the first data sample.
      |  4) Implement counters using DSP48Es to save resources.
      mask init: same as adc16_mytest/snap/a
      mask TypeOptions storage: bram | dram
      mask Callback storage: snapshot_callback();
      mask TypeOptions dram_dimm: 1 | 2 | 3 | 4
      mask TypeOptions dram_clock: 200 | 250 | 266 | 300 | 333
      mask TypeOptions data_width: 8 | 16 | 32 | 64 | 128
  g : Subsystem  Tag=casper:snapshot  AncestorBlock=casper_library_scopes/snapshot  mask(snapshot){storage=bram, dram_dimm=1, dram_clock=200, nsamples=10, data_width=32, offset=off, circap=off, value=off, use_dsp48=off}
      mask prompts: storage "Storage medium"; dram_dimm "DRAM dimm"; dram_clock "DRAM clock rate"; nsamples "Number of Samples (2^?)"; data_width "Data width"; offset "Start delay support"; circap "Circular capture support"; value "Extra value capture support"; use_dsp48 "Use DSP48s to implement counters"
      mask help:
      | Standard snap block, but with the following optional extras;
      |  1) Optionally delay the fabric trigger by a user-specified number of valids.
      |  2) Capture continuously after a trigger until a stop pulse is received. Data is captured into BRAM continuously, with old data being overwritten until a stop command is received. Then stop capturing when memory is filled. This enables you to get some data before and some data after the stop pulse. Use the 'tr_en_cnt' register to determine where you are in your vector. 'Addr' register's MSb now indicates 'busy capturing'.
      |  3) Optionally capture a value on an input port to a register at the same time as the first data sample.
      |  4) Implement counters using DSP48Es to save resources.
      mask init: same as adc16_mytest/snap/a
      mask TypeOptions storage: bram | dram
      mask Callback storage: snapshot_callback();
      mask TypeOptions dram_dimm: 1 | 2 | 3 | 4
      mask TypeOptions dram_clock: 200 | 250 | 266 | 300 | 333
      mask TypeOptions data_width: 8 | 16 | 32 | 64 | 128
  h : Subsystem  Tag=casper:snapshot  AncestorBlock=casper_library_scopes/snapshot  mask(snapshot){storage=bram, dram_dimm=1, dram_clock=200, nsamples=10, data_width=32, offset=off, circap=off, value=off, use_dsp48=off}
      mask prompts: storage "Storage medium"; dram_dimm "DRAM dimm"; dram_clock "DRAM clock rate"; nsamples "Number of Samples (2^?)"; data_width "Data width"; offset "Start delay support"; circap "Circular capture support"; value "Extra value capture support"; use_dsp48 "Use DSP48s to implement counters"
      mask help:
      | Standard snap block, but with the following optional extras;
      |  1) Optionally delay the fabric trigger by a user-specified number of valids.
      |  2) Capture continuously after a trigger until a stop pulse is received. Data is captured into BRAM continuously, with old data being overwritten until a stop command is received. Then stop capturing when memory is filled. This enables you to get some data before and some data after the stop pulse. Use the 'tr_en_cnt' register to determine where you are in your vector. 'Addr' register's MSb now indicates 'busy capturing'.
      |  3) Optionally capture a value on an input port to a register at the same time as the first data sample.
      |  4) Implement counters using DSP48Es to save resources.
      mask init: same as adc16_mytest/snap/a
      mask TypeOptions storage: bram | dram
      mask Callback storage: snapshot_callback();
      mask TypeOptions dram_dimm: 1 | 2 | 3 | 4
      mask TypeOptions dram_clock: 200 | 250 | 266 | 300 | 333
      mask TypeOptions data_width: 8 | 16 | 32 | 64 | 128
  wires:
  [adc_bus] -> Bus Selector2/1
  Bus Selector2/16 -> BitBasher11/4  "<h4>"
  Bus Selector2/15 -> BitBasher11/3  "<h3>"
  Bus Selector2/14 -> BitBasher11/2  "<h2>"
  Bus Selector2/13 -> BitBasher11/1  "<h1>"
  Bus Selector2/12 -> BitBasher10/4  "<g4>"
  Bus Selector2/11 -> BitBasher10/3  "<g3>"
  Bus Selector2/10 -> BitBasher10/2  "<g2>"
  Bus Selector2/9 -> BitBasher10/1  "<g1>"
  Bus Selector2/8 -> BitBasher9/4  "<f4>"
  Bus Selector2/7 -> BitBasher9/3  "<f3>"
  Bus Selector2/6 -> BitBasher9/2  "<f2>"
  Bus Selector2/5 -> BitBasher9/1  "<f1>"
  Bus Selector2/4 -> BitBasher8/4  "<e4>"
  Bus Selector2/3 -> BitBasher8/3  "<e3>"
  Bus Selector2/2 -> BitBasher8/2  "<e2>"
  Bus Selector2/1 -> BitBasher8/1  "<e1>"
  [adc_bus] -> Bus Selector/1
  Bus Selector/16 -> BitBasher3/4  "<d4>"
  Bus Selector/15 -> BitBasher3/3  "<d3>"
  Bus Selector/14 -> BitBasher3/2  "<d2>"
  Bus Selector/13 -> BitBasher3/1  "<d1>"
  Bus Selector/12 -> BitBasher2/4  "<c4>"
  Bus Selector/11 -> BitBasher2/3  "<c3>"
  Bus Selector/10 -> BitBasher2/2  "<c2>"
  Bus Selector/9 -> BitBasher2/1  "<c1>"
  Bus Selector/8 -> BitBasher1/4  "<b4>"
  Bus Selector/7 -> BitBasher1/3  "<b3>"
  Bus Selector/6 -> BitBasher1/2  "<b2>"
  Bus Selector/5 -> BitBasher1/1  "<b1>"
  Bus Selector/4 -> BitBasher/4  "<a4>"
  Bus Selector/3 -> BitBasher/3  "<a3>"
  Bus Selector/2 -> BitBasher/2  "<a2>"
  Bus Selector/1 -> BitBasher/1  "<a1>"
  BitBasher11/1 -> h/1(din)
  BitBasher10/1 -> g/1(din)
  BitBasher9/1 -> f/1(din)
  BitBasher8/1 -> e/1(din)
  Constant2/1 -> e/2(we), f/2(we), h/2(we), g/2(we)
  [trig] -> Slice/1
  BitBasher3/1 -> d/1(din)
  BitBasher2/1 -> c/1(din)
  BitBasher1/1 -> b/1(din)
  BitBasher/1 -> a/1(din)
  Slice/1 -> h/3(trig), g/3(trig), f/3(trig), e/3(trig), d/3(trig), c/3(trig), b/3(trig), a/3(trig)
  Constant1/1 -> a/2(we), b/2(we), d/2(we), c/2(we)

== system adc16_mytest/trig ==
  sim_1 : Inport
  adc16_mytest_trig_user_data_out : xbsIndex_r4/Gateway In  gui_display_data_type=Fixed-point  arith_type=Unsigned  n_bits=32  bin_pt=0  preci_type=Single  exp_width=8  frac_width=24  quantization="Round  (unbiased: +/- Inf)"  overflow=Saturate  period=1  dbl_ovrd=off  timing_constraint=None  locs_specified=off  LOCs={}  UseAsADC=off  ADCChannel='1'  inherit_from_input=off  hdl_port=on  block_type=gatewayin
  io_delay : xbsIndex_r4/Delay  rst=off  infoeditControl=Selection of Reset will increase slice count due to use of real FFs and instead of SRLs  en=off  latency=0  dbl_ovrd=off  reg_retiming=on  block_type=delay
  reint1 : xbsIndex_r4/Reinterpret  force_arith_type=on  arith_type=Unsigned  force_bin_pt=on  bin_pt=0  block_type=reinterpret
  slice_reg : xbsIndex_r4/Slice  nbits=32  boolean_output=off  mode=Lower Bit Location + Width  bit1=0  base1=MSB of Input  bit0=0  base0=LSB of Input  dbl_ovrd=off  block_type=slice
  in_reg : Outport
  wires:
  adc16_mytest_trig_user_data_out/1 -> io_delay/1
  sim_1/1 -> adc16_mytest_trig_user_data_out/1
  io_delay/1 -> slice_reg/1
  slice_reg/1 -> reint1/1
  reint1/1 -> in_reg/1
